simulink model "untitled"  (Simulink 7.7)
settings: Solver=ode45  StartTime=0.0  StopTime=2  FixedStep=100  RelTol=1e-3
values from neighbouring files (symbols this model uses):
  J = ((0.543)*(1000*100*100))    (= 5430000)    [parametriza_modelo_motorDc.m]
  k1 = -(((Ra)/(La))+((B)/(J)))    (= -28739.4957983)    [parametriza_modelo_motorDc.m]
  k2 = -((((Ra)*(B))+((alpha)^2))/((J)*(La)))    (= -2.80112044818e-05)    [parametriza_modelo_motorDc.m]
  k3 = ((alpha)/((J)*(La)))    (= 1.54758035811e-05)    [parametriza_modelo_motorDc.m]
  k4 = -((1)/(J))    (= -1.84162062615e-07)    [parametriza_modelo_motorDc.m]
  k5 = -((Ra)/((J)*(La)))    (= -0.00529272482474)    [parametriza_modelo_motorDc.m]
settings Model: Creator=Felipe  LastModifiedBy=Felipe
settings OptimizationCC: EfficientMapNaN2IntZero=off
settings HardwareCC: TargetIntDivRoundTo=Zero  TargetEndianess=LittleEndian  TargetHWDeviceType=MATLAB Host  ProdEqTarget=off
settings RTWCC: SystemTargetFile=accel.tlc  TemplateMakefile=accel_default_tmf  RTWVerbose=off  ProcessScript=accel_make_rtw_hook
settings CodeAppCC: MaxIdLength=128
settings STFCustomTargetCC: FunctionExecutionProfile=off  GeneratePreprocessorConditionals=Disable all  SystemTargetFile=accel.tlc

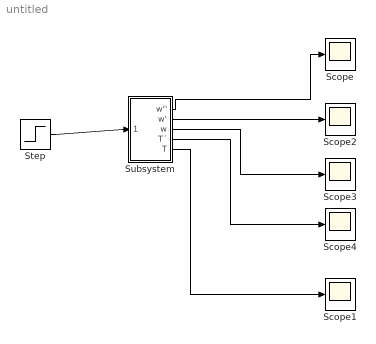
== system untitled ==
  Scope{,1..4} (5 alike) : Scope
      Scope settings: YMin=0.00025  YMax=0.003
      Scope2 settings: SaveName=ScopeData2
      Scope3 settings: SaveName=ScopeData3
      Scope4 settings: SaveName=ScopeData4
  Step : Step  SampleTime=0
  Subsystem : Subsystem
  wires:
  Step/1 -> Subsystem/1(e(t))
  Subsystem/1(w'') -> Scope/1
  Subsystem/5(T) -> Scope1/1
  Subsystem/2(w') -> Scope2/1
  Subsystem/3(w) -> Scope3/1
  Subsystem/4(T´) -> Scope4/1

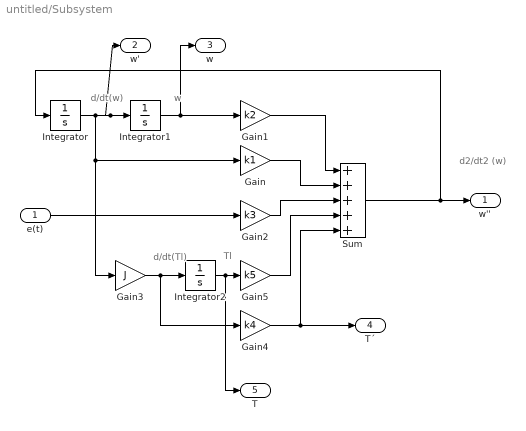
== system untitled/Subsystem ==
  note: w
  note: d/dt(w)
  note: d/dt(Tl)
  note: Tl
  note: d2/dt2 (w)
  e(t) : Inport
  Gain : Gain  Gain=k1
  Gain1 : Gain  Gain=k2
  Gain2 : Gain  Gain=k3
  Gain3 : Gain  Gain=J
  Gain4 : Gain  Gain=k4
  Gain5 : Gain  Gain=k5
  Integrator : Integrator
  Integrator1 : Integrator
  Integrator2 : Integrator
  Sum : Sum  Inputs=+++++
  w'' : Outport
  w' : Outport  Port=2
  w : Outport  Port=3
  T´ : Outport  Port=4
  T : Outport  Port=5
  wires:
  Integrator/1 -> Gain/1, Gain3/1, Integrator1/1, w'/1
  Integrator1/1 -> Gain1/1, w/1
  e(t)/1 -> Gain2/1
  Integrator2/1 -> T/1, Gain5/1
  Gain3/1 -> Integrator2/1, Gain4/1
  Gain4/1 -> Sum/5, T´/1
  Gain5/1 -> Sum/4
  Gain2/1 -> Sum/3
  Gain/1 -> Sum/2
  Gain1/1 -> Sum/1
  Sum/1 -> Integrator/1, w''/1
